simulink model "hbridge_lcl_grid_open_loop"  (R2025b)
settings: Solver=FixedStepDiscrete  StartTime=0.0  StopTime=T_sim_grid  FixedStep=T_step_grid  RelTol=1e-3
values from neighbouring files (symbols this model uses):
  m_sync = V_grid_pk/Vdc_grid    [grid_tie_params.m]
  m_test = m_sync + delta_m_test    [grid_tie_params.m]
  t_breaker = 0.080    (= 0.08)    [grid_tie_params.m]
  t_injection = 0.140    (= 0.14)    [grid_tie_params.m]
  V_grid_pk = sqrt(2)*V_grid_rms    [grid_tie_params.m]
  Vdc_grid = 48.0    (= 48)    [grid_tie_params.m]
  w_grid_tie = 2*pi*f_grid_tie    (= 314.159265359)    [grid_tie_params.m]
libraries: simulink x1
settings Model: Creator=hemanggadhvi  LastModifiedBy=hemanggadhvi

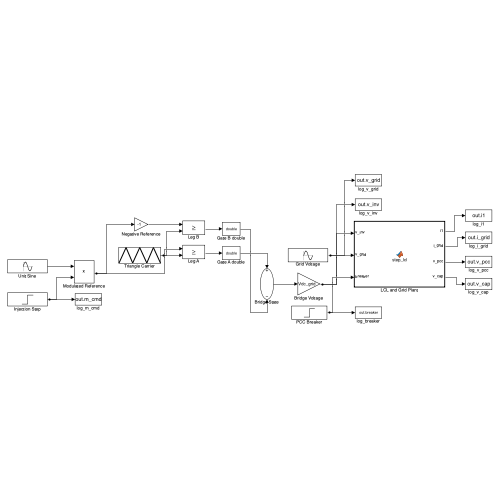
[thumbnail: Simulink's stored preview of the top-level diagram]
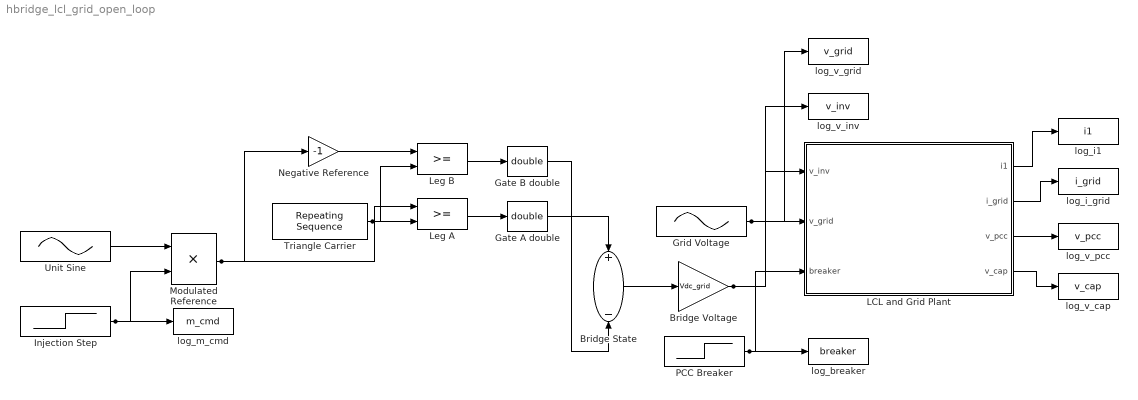
== system hbridge_lcl_grid_open_loop ==
  Bridge State : Sum  Inputs=+-
  Bridge Voltage : Gain  Gain=Vdc_grid
  Gate A double : DataTypeConversion  OutDataTypeStr=double  SaturateOnIntegerOverflow=off  RndMeth=Floor
  Gate B double : DataTypeConversion  OutDataTypeStr=double  SaturateOnIntegerOverflow=off  RndMeth=Floor
  Grid Voltage : Sin  Amplitude=V_grid_pk  Frequency=w_grid_tie  SampleTime=0
  Injection Step : Step  Time=t_injection  Before=m_sync  After=m_test  SampleTime=0
  LCL and Grid Plant : MATLAB Function  TreatAsAtomicUnit=on
  Leg A : RelationalOperator  OutDataTypeStr=boolean  RndMeth=Simplest  InputSameDT=off
  Leg B : RelationalOperator  OutDataTypeStr=boolean  RndMeth=Simplest  InputSameDT=off
  Modulated Reference : Product
  Negative Reference : Gain  Gain=-1
  PCC Breaker : Step  Time=t_breaker  SampleTime=0
  Triangle Carrier : simulink/Sources/Repeating Sequence  rep_seq_t=carrier_time_grid  rep_seq_y=carrier_values_grid
  Unit Sine : Sin  Frequency=w_grid_tie  SampleTime=0
  log_breaker : ToWorkspace  VariableName=breaker  SaveFormat=Timeseries  SampleTime=-1
  log_i1 : ToWorkspace  VariableName=i1  SaveFormat=Timeseries  SampleTime=-1
  log_i_grid : ToWorkspace  VariableName=i_grid  SaveFormat=Timeseries  SampleTime=-1
  log_m_cmd : ToWorkspace  VariableName=m_cmd  SaveFormat=Timeseries  SampleTime=-1
  log_v_cap : ToWorkspace  VariableName=v_cap  SaveFormat=Timeseries  SampleTime=-1
  log_v_grid : ToWorkspace  VariableName=v_grid  SaveFormat=Timeseries  SampleTime=-1
  log_v_inv : ToWorkspace  VariableName=v_inv  SaveFormat=Timeseries  SampleTime=-1
  log_v_pcc : ToWorkspace  VariableName=v_pcc  SaveFormat=Timeseries  SampleTime=-1
  wires:
  LCL and Grid Plant/4(v_cap) -> log_v_cap/1
  LCL and Grid Plant/2(i_grid) -> log_i_grid/1
  PCC Breaker/1 -> log_breaker/1, LCL and Grid Plant/3(breaker)
  LCL and Grid Plant/1(i1) -> log_i1/1
  Bridge State/1 -> Bridge Voltage/1
  Gate A double/1 -> Bridge State/1
  Gate B double/1 -> Bridge State/2
  Bridge Voltage/1 -> log_v_inv/1, LCL and Grid Plant/1(v_inv)
  Leg B/1 -> Gate B double/1
  Unit Sine/1 -> Modulated Reference/1
  Negative Reference/1 -> Leg B/1
  Modulated Reference/1 -> Negative Reference/1, Leg A/1
  LCL and Grid Plant/3(v_pcc) -> log_v_pcc/1
  Leg A/1 -> Gate A double/1
  Injection Step/1 -> log_m_cmd/1, Modulated Reference/2
  Grid Voltage/1 -> log_v_grid/1, LCL and Grid Plant/2(v_grid)
  Triangle Carrier/1 -> Leg B/2, Leg A/2

== matlab function hbridge_lcl_grid_open_loop/LCL and Grid Plant ==
  data: v_inv input; i1 output; v_grid input; breaker input; i_grid output; v_pcc output; v_cap output
function [i1,i_grid,v_pcc,v_cap] = step_lcl(v_inv,v_grid,breaker)
%#codegen
persistent x_i1 x_ig x_vc
if isempty(x_i1); x_i1=0; x_ig=0; x_vc=0; end
Ts=9.9999999999999995e-07; L1=0.00014999999999999999; R1=0.014999999999999999; C=2.0000000000000002e-05; Rd=0.56000000000000005; L2=9.4999999999999992e-05; R2=0.065000000000000002;
if breaker < 0.5; x_ig=0; end
i_cap=x_i1-x_ig; v_node=x_vc+Rd*i_cap;
di1=(v_inv-R1*x_i1-v_node)/L1;
dvc=i_cap/C;
if breaker >= 0.5; dig=(v_node-R2*x_ig-v_grid)/L2; else; dig=0; end
x_i1=x_i1+Ts*di1; x_vc=x_vc+Ts*dvc;
if breaker >= 0.5; x_ig=x_ig+Ts*dig; else; x_ig=0; end
i1=x_i1; i_grid=x_ig; v_cap=x_vc; v_pcc=x_vc+Rd*(x_i1-x_ig);
end
